simulink model "kadai31"  (R2021b)
settings: Solver=VariableStepAuto  StartTime=0.0  StopTime=8000  MaxStep=0.01  RelTol=1e-3
settings Model: Creator=tomotomo  LastModifiedBy=tomotomo

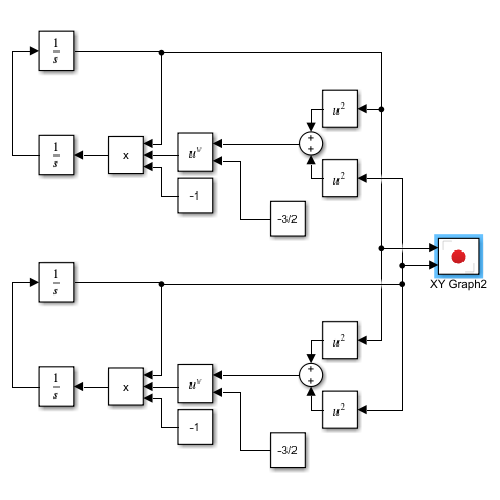
[thumbnail: Simulink's stored preview of the top-level diagram]
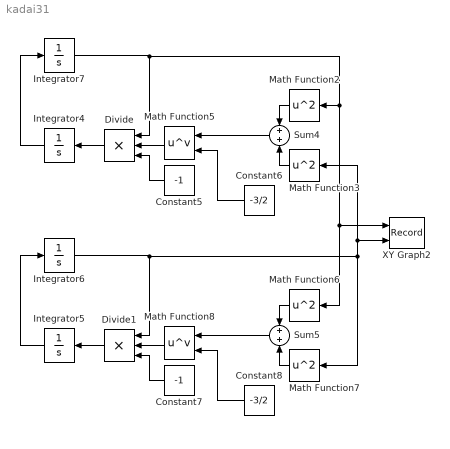
== system kadai31 ==
  Constant5 : Constant  Value=-1
  Constant6 : Constant  Value=-3/2
  Constant7 : Constant  Value=-1
  Constant8 : Constant  Value=-3/2
  Divide : Product  Inputs=***
  Divide1 : Product  Inputs=***
  Integrator4 : Integrator  InitialCondition=1.0
  Integrator5 : Integrator  InitialCondition=0.0
  Integrator6 : Integrator  InitialCondition=2.0
  Integrator7 : Integrator  InitialCondition=0.0
  Math Function{2..3,6..7} (4 alike) : Math  Operator=square  SaturateOnIntegerOverflow=on
  Math Function5 : Math  Operator=pow  SaturateOnIntegerOverflow=on
  Math Function8 : Math  Operator=pow  SaturateOnIntegerOverflow=on
  Sum4 : Sum  Inputs=+|+
  Sum5 : Sum  Inputs=+|+
  XY Graph2 : Record  FileSettingsInternal="{\"entries\":[{\"content\":{\"excelSettings\":{\"content\":{},\"type\":\"Streamout.ExcelSettings\"}},\"type\":\"Streamout.FileSettingStorage\",\"uuid\":\"7e2fcadf-ba1a-438c-8d67-a0e940803354\"}],\"packageUris\":[\"http://schema.mathworks.com/mf0/streamout_blocks/R2020a\"],\"version\":\"1.0\"}"  Layout=[1 1]  SignalsInternal="{\"entries\":[{\"content\":{\"signals\":[{\"content\":{\"blockPath\":[\"kadai31/XY Graph2\"],\"channel\":[],\"dimensions\":[1],\"domain\":\"kadai31/XY Graph2\",\"lineColor\":\"#a2142f\",\"plots\":[1],\"port\":1,\"sid\":[\"\"],\"signalID\":11103,\"signalName\":\"Integrator7\"},\"type\":\"RecordBlkView.Signal\",\"uuid\":\"ff0407ae-f339-4f03-b460-e06ca502a65b\"},{\"content\":{\"blockPath\":[\"kadai31/XY Graph2\"],\"channel\":[],\"dimensions\":[1],\"domain\":\"kadai31/XY Graph2\",\"lineColor\":\"#139fff\",\"plots\":[1],\"port\":2,\"sid\":[\"\"],\"signalID\":11107,\"signalName\":\"Integrator6\"},\"type\":\"RecordBlkView.Signal\",\"uuid\":\"8c3508c7-6d79-46b7-9a85-b6fa65f3e956\"}]},\"type\":\"RecordBlkView.InputSignals\",\"uuid\":\"6703c3a8-ace4-4b1e-beca-a69b89a401e9\"}],\"packageUris\":[\"http://schema.mathworks.com/mf0/streamout_blocks/R2020a\"],\"version\":\"1.0\"}"  VisualizationBindings="{\"xyplotplugin\":{\"info\":[{\"series\":[{\"bindingParametersList\":[{\"parameter\":\"X-Axis\",\"signalID\":11103,\"signalName\":\"Integrator7\"},{\"parameter\":\"Y-Axis\",\"signalID\":11107,\"signalName\":\"Integrator6\"}],\"seriesID\":11102}],\"subplotID\":1}]}}"  CompatibilityTag=XY
  wires:
  Math Function2/1 -> Sum4/1
  Sum4/1 -> Math Function5/1
  Math Function3/1 -> Sum4/2
  Math Function5/1 -> Divide/2
  Constant6/1 -> Math Function5/2
  Divide/1 -> Integrator4/1
  Integrator4/1 -> Integrator7/1
  Constant5/1 -> Divide/3
  Constant8/1 -> Math Function8/2
  Divide1/1 -> Integrator5/1
  Math Function8/1 -> Divide1/2
  Constant7/1 -> Divide1/3
  Integrator5/1 -> Integrator6/1
  Math Function6/1 -> Sum5/1
  Math Function7/1 -> Sum5/2
  Sum5/1 -> Math Function8/1
  Integrator6/1 -> Divide1/1, Math Function3/1, XY Graph2/2, Math Function7/1
  Integrator7/1 -> Divide/1, Math Function6/1, XY Graph2/1, Math Function2/1
